simulink model "sldemo_absbrake"  (R2025b)
settings: Solver=ode45  StartTime=0.0  StopTime=22  FixedStep=0.01  MaxStep=.01  RelTol=1e-3  AbsTol=1e-6
PreLoadFcn:
  | % Load initialization data
  | 
  | sldemo_absdata;
  | mu_dry = mu;
  | mu_wet = mu * 0.5;
  | mu_ice = mu * 0.15;
StopFcn:
  |  if exist ('sldemo_absbrake_output')
  |  sldemo_absbrakeplots;
  |  end
values from neighbouring files (symbols this model uses):
  ctrl = 0    [ModelingAnAntiLockBrakingSystemExample.m]    (also in m.mat = 1; mu.mat = 1; mu_values.mat = 1)
  g = 32.18    [m.mat]    (also in mu.mat; mu_values.mat)
  m = 50    [m.mat]    (also in mu.mat; mu_values.mat)
  mu = [0 0.4 0.8 0.97 1 0.98 0.96 0.94 0.92 0.9 0.88 0.855 ... (21 elements, 1x21)]    [m.mat]    (also in mu.mat; mu_values.mat)
  Rr = 1.25    [m.mat]    (also in mu.mat; mu_values.mat)
  slip = [0 0.05 0.1 0.15 0.2 0.25 0.3 0.35 0.4 0.45 0.5 0.55 ... (21 elements, 1x21)]    [m.mat]    (also in mu.mat; mu_values.mat)
  v0 = 88    [m.mat]    (also in mu.mat; mu_values.mat)
undefined symbols (not defined in the file or in its folder): DiscIntNeverNeededParam
libraries: simulink x1, simulink_extras x1
CloseFcn:
  | % Close the plots that are still open
  | h = findobj(0, 'Name', 'ABS Speeds');
  | if ~isempty(h),
  |   close(h);
  | end;
  | 
  | h = findobj(0, 'Name', 'ABS Slip');
  | if ~isempty(h),
  |   close(h);
  | end;
  | 
  | % Clear initial conditions data to avoid cluttering the workspace
  | 
  | clear g v0 Rr Kf m PBmax TB I slip mu ctrl h;
Description:
  | Modeling an Anti-Lock Braking System (ABS)
  | 
  | *Summary*
  | 
  | This example describes a simple model for an Anti-Lock Braking System
  | (ABS). The model simulates the dynamic behavior of a vehicle
  | under hard braking conditions. The model represents a single wheel, which
  | may be replicated a number of times to create a model for a multi-wheel
  | vehicle.
  | 
  | This model uses the signal logging feature in Simulink(R). You log signals to the
  | MATLAB(R) workspace where you can analyze and view them. You can view
  | the code in sldemo_absbrakeplots.m to see how this is done.
  | 
  | In this model, the wheel speed is calculated in a separate component
  | named sldemo_wheelspeed_absbrake.
  | This component is then referenced using a Model block.  Note that both the
  | top model and the referenced model use a variable step solver, so Simulink
  | will track zero-crossings in the referenced model.
settings Model: FPTRunName=Active  ModifiedByFormat=The MathWorks, Inc.  SILPILSystemUnderTest=refmodels  CodeVerificationMode=processor-in-the-loop (pil)  ExtModeTrigMode=oneshot  ExtModeArmWhenConnect=off  ExtModeAutoUpdateStatusClock=off  Creator=The MathWorks, Inc.  LastModifiedBy=The MathWorks, Inc.
settings SolverCC: AutoScaleAbsTol=off  AlgebraicLoopSolver=TrustRegion  MaxZcPerStep=1.0
settings DataIOCC: SaveTime=off  ReturnWorkspaceOutputs=off  TimeSaveName=time
settings OptimizationCC: DefaultParameterBehavior=Inlined  UseDivisionForNetSlopeComputation=on  InlineInvariantSignals=on  EnhancedBackFolding=on  PassReuseOutputArgsAs=Individual arguments  ExpressionDepthLimit=2147483647.0  StateBitsets=on  DataBitsets=on  ZeroExternalMemoryAtStartup=off  ZeroInternalMemoryAtStartup=off  EfficientFloat2IntCast=on  LifeSpan=inf  MaxStackSize=64  BufferReusableBoundary=off  OptimizeBlockOrder=speed  DifferentSizesBufferReuse=on  EfficientTunableParamExpr=on
settings DebuggingCC: SignalInfNanChecking=warning  SaveWithParameterizedLinksMsg=none  SigSpecEnsureSampleTimeMsg=none  IntegerOverflowMsg=error  ParameterTunabilityLossMsg=error  UnconnectedInputMsg=warning  UnconnectedOutputMsg=warning  UnconnectedLineMsg=warning  UniqueDataStoreMsg=error  BusObjectLabelMismatch=none  AssertControl=DisableAll  AllowSymbolicDim=off  StateNameClashWarn=warning  SubsystemReferenceDiagnosticForUnitTest=warning  SFUnexpectedBacktrackingDiag=warning  SFNoUnconditionalDefaultTransitionDiag=warning  SFUndirectedBroadcastEventsDiag=error  SFExecutionAtInitializationDiag=none  IntegerSaturationMsg=none  ArithmeticOperatorsInVariantConditions=warning
settings HardwareCC: ProdBitPerPointer=32.0  ProdBitPerSizeT=32.0  ProdBitPerPtrDiffT=32.0  ProdLargestAtomicInteger=Long  ProdLargestAtomicFloat=Double  ProdWordSize=32.0  ProdHWDeviceType=ARM Compatible->ARM Cortex  TargetBitPerPointer=64.0  TargetBitPerSizeT=64.0  TargetBitPerPtrDiffT=64.0  TargetLongLongMode=on  TargetIntDivRoundTo=Zero  TargetEndianess=LittleEndian  TargetWordSize=64.0  TargetHWDeviceType=MATLAB Host
settings ModelReferenceCC: UpdateModelReferenceTargets=IfOutOfDate  EnableRefExpFcnMdlSchedulingChecks=on  PropagateSignalLabelsOutOfModel=off
settings SFSimCC: SimUseLocalCustomCode=off  CompileTimeRecursionLimit=0.0  EnableRuntimeRecursion=off  MATLABDynamicMemAlloc=off  CustomCodeUndefinedFunction=UseInterfaceOnly
settings RTWCC: SystemTargetFile=ert.tlc  HardwareBoard=Arm Cortex-M7 Fast Model  TemplateMakefile=ert_default_tmf  RTWUseLocalCustomCode=off  Toolchain=GNU Tools for ARM Embedded Processors  CodeProfilingSaveOptions=AllData  CodeProfilingInstrumentation=detailed  GPUComputeCapability=3.5  DLArmComputeVersion=19.05  Description=Embedded Coder
settings CodeAppCC: ForceParamTrailComments=on  IgnoreCustomStorageClasses=off  IgnoreTestpoints=on  OperatorAnnotations=on  SimulinkDataObjDesc=on  SFDataObjDesc=on  MATLABFcnDesc=on  InsertBlockDesc=on
settings ERTTargetCC: SuppressUnreachableDefaultCases=off  EnableSignedLeftShifts=off  EnableSignedRightShifts=off  DynamicArrayContainerType=coder::array  UtilityFuncGeneration=Shared location  SupportAbsoluteTime=off  ParenthesesLevel=Standards  CastingMode=Standards  GenerateSharedConstants=off
settings ConfigComp: CovEnable=on  CovScope=ReferencedModels  RecordCoverage=on  CovMetricSettings=dcmw  CovSaveCumulativeToWorkspaceVar=on  CovSaveSingleToWorkspaceVar=on  CovCumulativeVarName=covdata  CovModelRefEnable=filtered  CovExternalEMLEnable=off  CovSFcnEnable=off

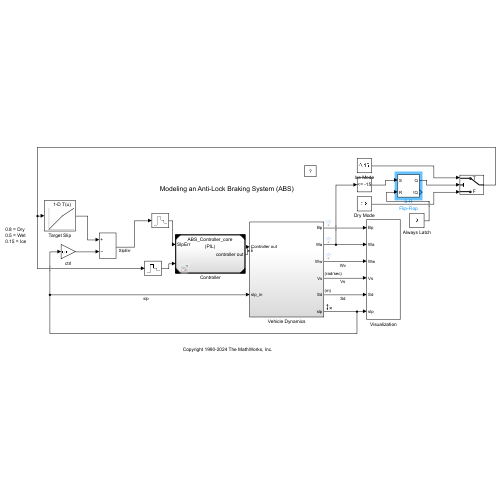
[thumbnail: Simulink's stored preview of the top-level diagram]
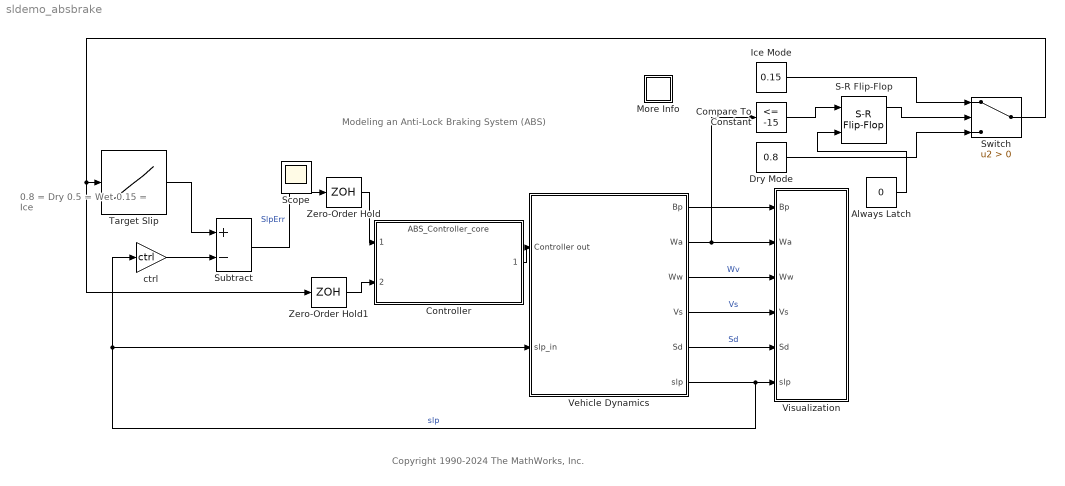
== system sldemo_absbrake ==
  note: 0.8 = Dry
      | 0.5 = Wet
      | 0.15 = Ice
  note: Modeling an Anti-Lock Braking System (ABS)
  note: Copyright 1990-2024 The MathWorks, Inc.
  Always Latch : Constant  Value=0  OutDataTypeStr=boolean
  Compare To Constant : simulink/Logic and Bit Operations/Compare To Constant  relop=<=  const=-15  OutDataTypeStr=boolean
  Controller : ModelReference  ModelNameDialog=ABS_Controller_core  SimulationMode=Processor-in-the-loop (PIL)  ModelReferenceVersion=11.15
  Dry Mode : Constant  Value=0.8
  Ice Mode : Constant  Value=0.15
  More Info : Subsystem
      settings: OpenFcn=showExample('simulink_automotive/ModelingAnAntiLockBrakingSystemExample')
      mask Display: disp('?')
  S-R Flip-Flop : simulink_extras/Flip Flops/S-R Flip-Flop  initial_condition=0
  Subtract : Sum  Inputs=+-
  Switch : Switch  Criteria=u2 > Threshold  SaturateOnIntegerOverflow=off  InputSameDT=off
  Target Slip : Lookup_n-D  NumberOfTableDimensions=1  BreakpointsForDimension1=[0.15,0.5,0.8]  Table=[0.065,0.15,0.2]  InternalRulePriority=Speed  RndMeth=Simplest
  Vehicle Dynamics : Subsystem
  Visualization : Subsystem
  Zero-Order Hold : ZeroOrderHold  SampleTime=0.01
  Zero-Order Hold1 : ZeroOrderHold  SampleTime=0.01
  ctrl : Gain  Gain=ctrl
  Scope : Scope
      settings: ActiveDisplayYMinimum=-8.8  ActiveDisplayYMaximum=79.2
  wires:
  Subtract/1 -> Zero-Order Hold/1  "SlpErr"
  Target Slip/1 -> Subtract/1
  ctrl/1 -> Subtract/2
  Vehicle Dynamics/6(slp) -> ctrl/1, Vehicle Dynamics/2(slp_in), Visualization/6(slp)  "slp"
  Controller/1 -> Vehicle Dynamics/1(Controller out)
  Vehicle Dynamics/1(Bp) -> Visualization/1(Bp)
  Vehicle Dynamics/2(Wa) -> Compare To Constant/1, Visualization/2(Wa)
  Vehicle Dynamics/3(Ww) -> Visualization/3(Ww)  "Wv"
  Vehicle Dynamics/4(Vs) -> Visualization/4(Vs)  "Vs"
  Vehicle Dynamics/5(Sd) -> Visualization/5(Sd)  "Sd"
  Switch/1 -> Zero-Order Hold1/1, Target Slip/1
  Dry Mode/1 -> Switch/3
  Ice Mode/1 -> Switch/1
  S-R Flip-Flop/1 -> Switch/2
  Compare To Constant/1 -> S-R Flip-Flop/1
  Always Latch/1 -> S-R Flip-Flop/2
  Zero-Order Hold/1 -> Controller/1
  Zero-Order Hold1/1 -> Controller/2

== system sldemo_absbrake/More Info ==

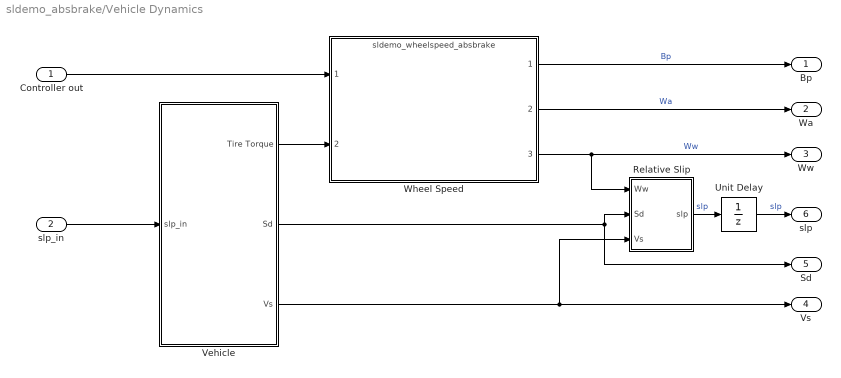
== system sldemo_absbrake/Vehicle Dynamics ==
  Controller out : Inport
  slp_in : Inport  Port=2
  Relative Slip : Subsystem
  Unit Delay : UnitDelay  SampleTime=-1  HasFrameUpgradeWarning=on
  Vehicle : Subsystem
  Wheel Speed : ModelReference  ModelNameDialog=sldemo_wheelspeed_absbrake.slx  SimulationMode=Normal  ModelReferenceVersion=11.1
  Bp : Outport
  Wa : Outport  Port=2
  Ww : Outport  Port=3
  Vs : Outport  Port=4
  Sd : Outport  Port=5
  slp : Outport  Port=6
  wires:
  Wheel Speed/3 -> Relative Slip/1(Ww), Ww/1  "Ww"
  Vehicle/3(Vs) -> Relative Slip/3(Vs), Vs/1
  Vehicle/1(Tire Torque) -> Wheel Speed/2
  Vehicle/2(Sd) -> Sd/1, Relative Slip/2(Sd)
  Relative Slip/1(slp) -> Unit Delay/1  "slp"
  Controller out/1 -> Wheel Speed/1
  Wheel Speed/1 -> Bp/1  "Bp"
  slp_in/1 -> Vehicle/1(slp_in)
  Wheel Speed/2 -> Wa/1  "Wa"
  Unit Delay/1 -> slp/1  "slp"

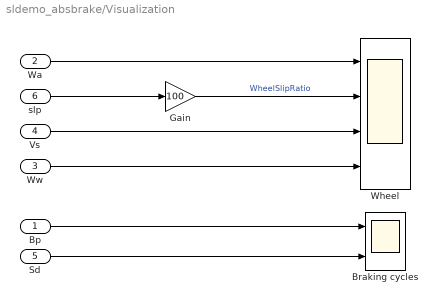
== system sldemo_absbrake/Visualization ==
  Bp : Inport
  Wa : Inport  Port=2
  Ww : Inport  Port=3
  Vs : Inport  Port=4
  Sd : Inport  Port=5
  slp : Inport  Port=6
  Braking cycles : Scope  NumInputPorts=2
      settings: ActiveDisplayYMinimum=-90.25511  ActiveDisplayYMaximum=812.29596
  Gain : Gain  Gain=100
  Wheel : Scope  NumInputPorts=4
      settings: ActiveDisplayYMinimum=-27.40083  ActiveDisplayYMaximum=12.545
  wires:
  Bp/1 -> Braking cycles/1
  Wa/1 -> Wheel/1
  Ww/1 -> Wheel/4
  Sd/1 -> Braking cycles/2
  Vs/1 -> Wheel/3
  Gain/1 -> Wheel/2  "WheelSlipRatio"
  slp/1 -> Gain/1

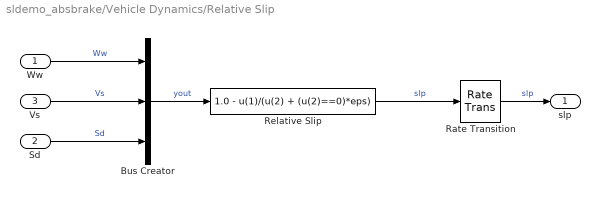
== system sldemo_absbrake/Vehicle Dynamics/Relative Slip ==
  Ww : Inport
  Sd : Inport  Port=2
  Vs : Inport  Port=3
  Bus Creator : BusCreator  Inputs=3
  Rate Transition : RateTransition  OutPortSampleTimeOpt=Inherit
  Relative Slip : Fcn  Expr=1.0 - u(1)/(u(2) + (u(2)==0)*eps)
  slp : Outport
  wires:
  Bus Creator/1 -> Relative Slip/1  "yout"
  Relative Slip/1 -> Rate Transition/1  "slp"
  Ww/1 -> Bus Creator/1  "Ww"
  Vs/1 -> Bus Creator/2  "Vs"
  Sd/1 -> Bus Creator/3  "Sd"
  Rate Transition/1 -> slp/1  "slp"

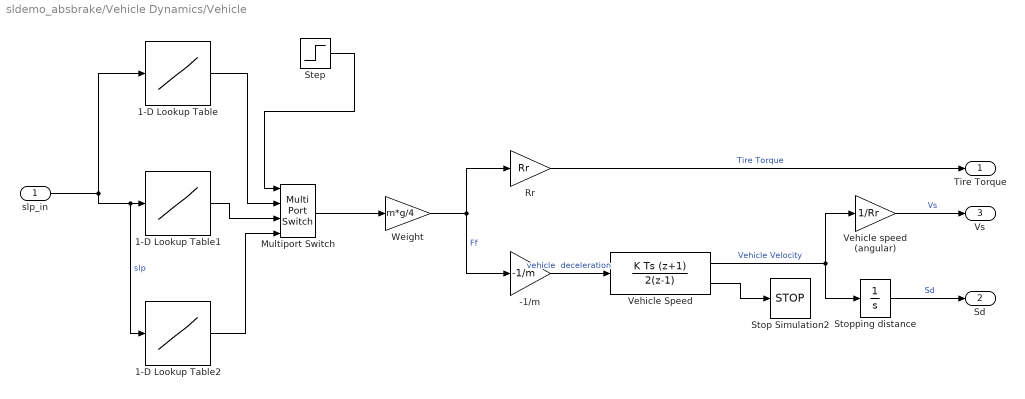
== system sldemo_absbrake/Vehicle Dynamics/Vehicle ==
  slp_in : Inport
  -1/m : Gain  Gain=-1/m  SaturateOnIntegerOverflow=on  OutDataTypeStr=Inherit: Same as input  ParamDataTypeStr=Inherit: Same as input
  1-D Lookup Table : Lookup_n-D  NumberOfTableDimensions=1  BreakpointsForDimension1=slip  Table=mu_dry  InternalRulePriority=Speed  RndMeth=Simplest
  1-D Lookup Table1 : Lookup_n-D  NumberOfTableDimensions=1  BreakpointsForDimension1=slip  Table=mu_wet  InternalRulePriority=Speed  RndMeth=Simplest
  1-D Lookup Table2 : Lookup_n-D  NumberOfTableDimensions=1  BreakpointsForDimension1=slip  Table=mu_ice  InternalRulePriority=Speed  RndMeth=Simplest
  Multiport Switch : MultiPortSwitch  SaturateOnIntegerOverflow=off  InputSameDT=off
  Rr : Gain  Gain=Rr  SaturateOnIntegerOverflow=on  OutDataTypeStr=Inherit: Same as input  ParamDataTypeStr=Inherit: Same as input
  Step : Step  Time=01  Before=1  SampleTime=0
  Stop Simulation2 : Stop
  Stopping distance : Integrator  UpperSaturationLimit=1000  LowerSaturationLimit=0
  Vehicle Speed : DiscreteIntegrator  IntegratorMethod=Integration: Trapezoidal  InitialCondition=v0  SampleTime=-1  LimitOutput=on  UpperSaturationLimit=1000  LowerSaturationLimit=0  ShowSaturationPort=on  ICPrevOutput=DiscIntNeverNeededParam  ICPrevScaledInput=DiscIntNeverNeededParam
  Vehicle speed (angular) : Gain  Gain=1/Rr  SaturateOnIntegerOverflow=on  OutDataTypeStr=Inherit: Same as input  ParamDataTypeStr=Inherit: Same as input
  Weight : Gain  Gain=m*g/4  SaturateOnIntegerOverflow=on  OutDataTypeStr=Inherit: Same as input  ParamDataTypeStr=Inherit: Same as input
  Tire Torque : Outport  Unit=N*m
  Sd : Outport  Port=2  Unit=m
  Vs : Outport  Port=3  Unit=rad/sec
  wires:
  Rr/1 -> Tire Torque/1  "Tire Torque"
  -1/m/1 -> Vehicle Speed/1  "vehicle  deceleration"
  Vehicle speed (angular)/1 -> Vs/1  "Vs"
  Stopping distance/1 -> Sd/1  "Sd"
  Weight/1 -> -1/m/1, Rr/1  "Ff"
  Vehicle Speed/1 -> Vehicle speed (angular)/1, Stopping distance/1  "Vehicle Velocity"
  Vehicle Speed/2 -> Stop Simulation2/1
  Multiport Switch/1 -> Weight/1
  1-D Lookup Table/1 -> Multiport Switch/2
  1-D Lookup Table1/1 -> Multiport Switch/3
  1-D Lookup Table2/1 -> Multiport Switch/4
  slp_in/1 -> 1-D Lookup Table2/1, 1-D Lookup Table1/1, 1-D Lookup Table/1  "slp"
  Step/1 -> Multiport Switch/1
